simulink model "python_control"  (R2025b)
settings: Solver=FixedStepAuto  StartTime=0.0  StopTime=5.0  RelTol=1e-3  EnableMultiTasking=on
settings Model: ExtModeTrigDuration=2  Creator=atcushen  LastModifiedBy=atcushen
settings SolverCC: PositivePriorityOrder=on
settings OptimizationCC: EnhancedBackFolding=on  PassReuseOutputArgsAs=Individual arguments  ZeroExternalMemoryAtStartup=off  ZeroInternalMemoryAtStartup=off  MaxStackSize=200000  OptimizeBlockOrder=speed  DifferentSizesBufferReuse=on  OptimizationCustomize=off  EfficientTunableParamExpr=on
settings DebuggingCC: ParameterTunabilityLossMsg=error
settings HardwareCC: ProdBitPerPointer=32.0  ProdBitPerSizeT=32.0  ProdBitPerPtrDiffT=32.0  ProdLargestAtomicInteger=Long  ProdLargestAtomicFloat=Double  ProdWordSize=32.0  ProdLongLongMode=on  ProdHWDeviceType=ARM Compatible->ARM Cortex-A (32-bit)  UseEmbeddedCoderFeatures=off  UseSimulinkCoderFeatures=off
settings RTWCC: SystemTargetFile=ert.tlc  HardwareBoard=Raspberry Pi  TLCOptions="-aInlineSetEventsForThisBaseRateFcn=TLC_FALSE -aSuppressMultiTaskScheduler=TLC_FALSE  -aRateBasedStepFcn=0"  TemplateMakefile=ert_default_tmf  Toolchain=GNU GCC Embedded Linux  BuildConfiguration=Faster Runs  Description=Embedded Coder
settings CodeAppCC: ForceParamTrailComments=on  IgnoreCustomStorageClasses=off  OperatorAnnotations=on  SimulinkDataObjDesc=on  SFDataObjDesc=on  MangleLength=10.0  InsertBlockDesc=on
settings ERTTargetCC: ExtModeTransport=2.0  ExtModeStaticAlloc=on  ExtModeMexFile=ext_xcp  ExtModeIntrfLevel=Level2 - Open  InlinedParameterPlacement=Hierarchical  SupportNonInlinedSFcns=on  SupportVariableSizeSignals=on

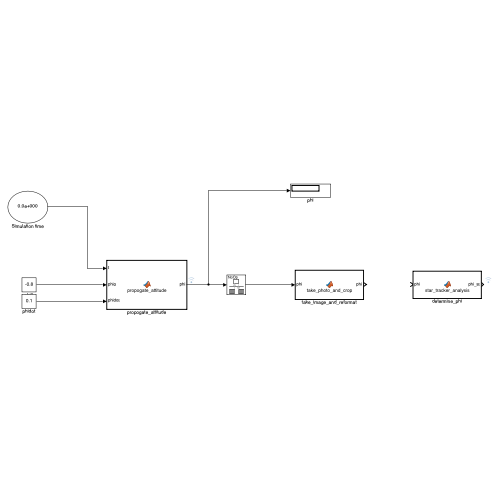
[thumbnail: Simulink's stored preview of the top-level diagram]
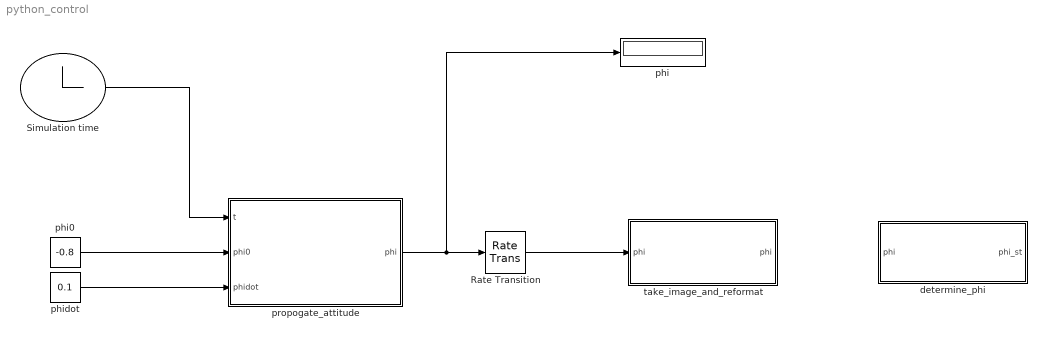
== system python_control ==
  Rate Transition : RateTransition  OutPortSampleTime=1
  Simulation time : Clock
  determine_phi : MATLAB Function  TreatAsAtomicUnit=on
  phi : Display
  phi0 : Constant  Value=-0.8
  phidot : Constant  Value=0.1
  propogate_attitude : MATLAB Function  TreatAsAtomicUnit=on
  take_image_and_reformat : MATLAB Function  TreatAsAtomicUnit=on
  wires:
  phidot/1 -> propogate_attitude/3(phidot)
  phi0/1 -> propogate_attitude/2(phi0)
  propogate_attitude/1(phi) -> phi/1, Rate Transition/1
  Simulation time/1 -> propogate_attitude/1(t)
  Rate Transition/1 -> take_image_and_reformat/1("phi ")

== matlab function python_control/determine_phi ==
  data: phi input; phi_st output
function phi_st = star_tracker_analysis(phi)
    
    root = "/home/space584a/MATLAB_ws/R2025b/";

    % Run analysis script
    cmd = 'python3 '+root+'ADCS_python/star_tracker.py';
    status = system(cmd);
    
    % Load the result
    struct = coder.load('ADCS_python/phi_st.mat');
    phi_st = struct.phi_st;
end

== matlab function python_control/take_image_and_reformat ==
  data: phi input; phi output
function phi = take_photo_and_crop(phi)
    
    root = "/home/space584a/MATLAB_ws/R2025b/";
    
    % Take photo
    shutter_time = 0.05; % [s]
    shutter_str = string(round(shutter_time * 1000000));
    cmd = 'sudo rpicam-still -o '+root+'ADCS_python/star_field.jpg --shutter '+shutter_str+' --gain 1 --awbgains 1,1 --immediate';
    %status = system(cmd);

    % Convert to cropped .npy
    cmd = 'python3 '+root+'ADCS_python/crop_image.py '+root+'ADCS_python/star_field.jpg';
    status = system(cmd);

    phi = phi; % Output the status or any other relevant information
end

== matlab function python_control/propogate_attitude ==
  data: t input; phi output; phi0 input; phidot input
% propogate attitude
function phi = propogate_attitude(t,phi0,phidot)
    % Input: 
    % t: float, current time, in s
    % phi0: float, initial attitude, in radians
    % phidot: float, rotation rate, in rad/sec
    
    % Output:
    % phi: float, current attitude, in rad/sec

    phi = mod(t*phidot + phi0 + pi,2*pi) - pi;
    %disp(['Propogated attitude at t = ',num2str(t),' to phi = ',num2str(phi)]);
end
